simulink model "DCMotorControlSheild_major"  (R2017a)
settings: Solver=VariableStepAuto  StartTime=0.0  StopTime=1.0  RelTol=1e-3
values from neighbouring files (symbols this model uses):
  Jm = 0.0000005    (= 5e-07)    [DCMotorControlSheild_sim.m]
  Kem = 0.001574    [DCMotorControlSheild_sim.m]
  Ktm = 0.001159    [DCMotorControlSheild_sim.m]
  Lm = 0.000340    (= 0.00034)    [DCMotorControlSheild_sim.m]
  Rm = 0.6818    [DCMotorControlSheild_sim.m]
settings Model: Creator=fumihiko  LastModifiedBy=fumihiko

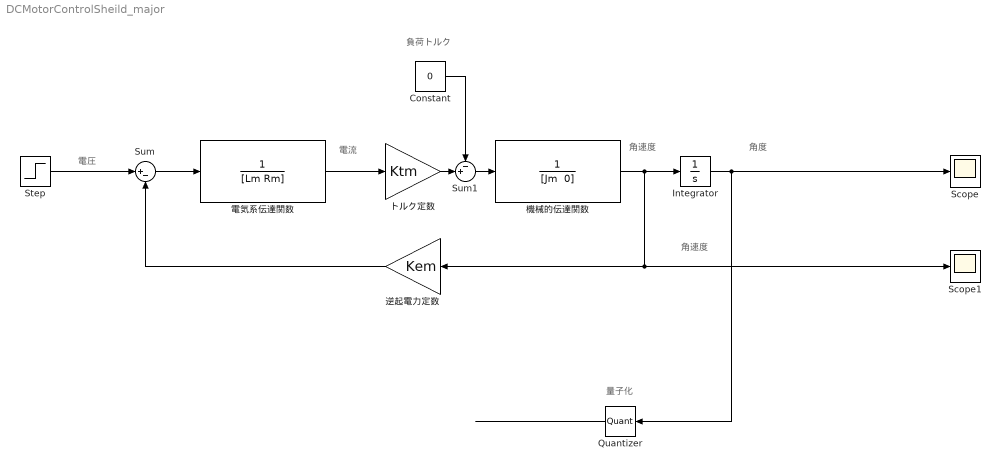
== system DCMotorControlSheild_major ==
  note: 電圧
  note: 角度
  note: 電流
  note: 負荷トルク
  note: 角速度
  note: 角速度
  note: 量子化
  Constant : Constant  Value=0
  Integrator : Integrator
  Quantizer : Quantizer  QuantizationInterval=dt_major
  Scope : Scope
  Scope1 : Scope
  Step : Step  Time=0.5  After=3.0  SampleTime=0
  Sum : Sum  Inputs=|+-
  Sum1 : Sum  Inputs=-+|
  トルク定数 : Gain  Gain=Ktm
  機械的伝達関数 : TransferFcn  Denominator="[Jm  0]"
  逆起電力定数 : Gain  Gain=Kem
  電気系伝達関数 : TransferFcn  Denominator=[Lm Rm]
  wires:
  電気系伝達関数/1 -> トルク定数/1
  Integrator/1 -> Quantizer/1, Scope/1
  機械的伝達関数/1 -> Integrator/1, Scope1/1, 逆起電力定数/1
  逆起電力定数/1 -> Sum/2
  Sum/1 -> 電気系伝達関数/1
  Step/1 -> Sum/1
  トルク定数/1 -> Sum1/2
  Sum1/1 -> 機械的伝達関数/1
  Constant/1 -> Sum1/1
  Quantizer/1 -> ?
